simulink model "DCM_Controller_Due"  (R2020a)
settings: Solver=FixedStepAuto  StartTime=0.0  StopTime=inf  FixedStep=T  RelTol=1e-3  EnableMultiTasking=on
undefined symbols (not defined in the file): Iumax, Ki_I, Kp_I, Kp_W, Kphi, T, Ubat, wmax
libraries: arduinolib x7, eeStairGenerator x2
settings Model: SILPILModeSetting=veronly  ExtModeTrigDuration=2  Creator=Nguyen Tung  LastModifiedBy=Nguyen Tung
settings OptimizationCC: StrengthReduction=on  PassReuseOutputArgsAs=Individual arguments  ZeroExternalMemoryAtStartup=off  ZeroInternalMemoryAtStartup=off  MaxStackSize=64  OptimizeBlockOrder=speed  OptimizationPriority=Speed  OptimizationCustomize=off  MultiThreadedLoops=on  EfficientTunableParamExpr=on
settings DebuggingCC: ParameterTunabilityLossMsg=error
settings HardwareCC: ProdBitPerPointer=32  ProdBitPerSizeT=32  ProdBitPerPtrDiffT=32  ProdLargestAtomicInteger=Long  ProdLargestAtomicFloat=Double  ProdWordSize=32  ProdHWDeviceType=ARM Compatible->ARM Cortex
settings SFSimCC: MATLABDynamicMemAlloc=off
settings RTWCC: SystemTargetFile=ert.tlc  HardwareBoard=Arduino Due  TLCOptions=-aInlineSetEventsForThisBaseRateFcn=TLC_FALSE -aSuppressMultiTaskScheduler=TLC_FALSE -aRateBasedStepFcn=1  TemplateMakefile=ert_default_tmf  GenerateReport=on  Toolchain=Arduino ARM  BuildConfiguration=Faster Runs
settings CodeAppCC: ForceParamTrailComments=on  IgnoreCustomStorageClasses=off  OperatorAnnotations=on  SimulinkDataObjDesc=on  SFDataObjDesc=on  InsertBlockDesc=on
settings ERTTargetCC: SupportContinuousTime=on  SupportVariableSizeSignals=on  ExtModeStaticAllocSize=20000

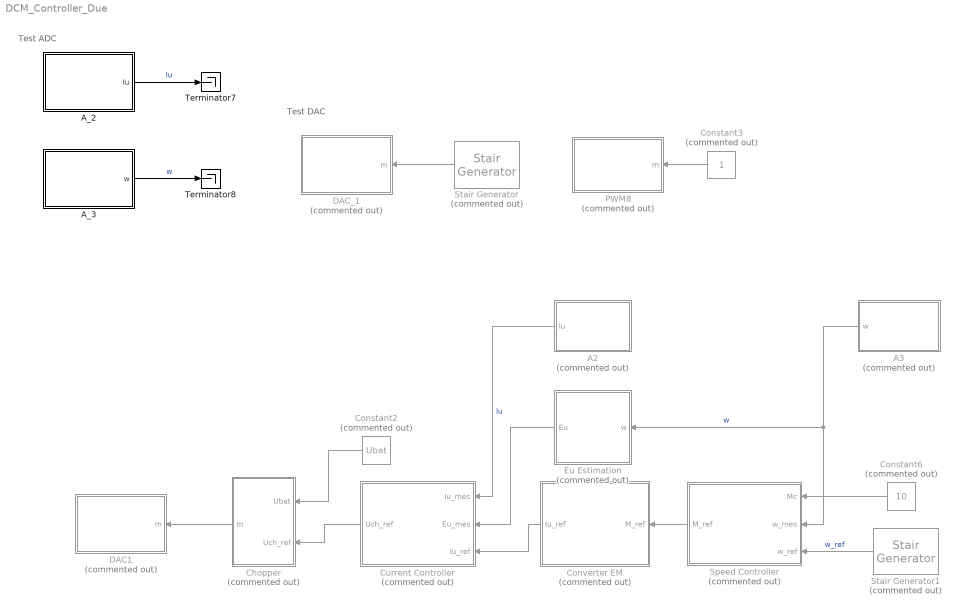
== system DCM_Controller_Due ==
  note: Test ADC
  note: Test DAC
  A2 : Subsystem  Commented=on
  A3 : Subsystem  Commented=on
  A_2 : Subsystem
  A_3 : Subsystem
  Chopper : Subsystem  Commented=on  AncestorBlock=simulink/SMC/Inversion EC avec mesure
      mask Display: plot(0,0,100,100,[10,30,90,70,10],[90,10,10,90,90])
  Constant2 : Constant  Commented=on  Value=Ubat
  Constant3 : Constant  Commented=on
  Constant6 : Constant  Commented=on  Value=10
  Converter EM : Subsystem  Commented=on  AncestorBlock=simulink/SMC/Inversion EC avec mesure
      mask Display: plot(0,0,100,100,[10,30,90,70,10],[90,10,10,90,90])
  Current Controller : Subsystem  Commented=on  AncestorBlock=simulink/SMC/Asservissement Correcteur IP
      mask Display: plot(0,0,100,100, [10,30,90,70,10,90],[90,10,10,90,90,10])
  DAC1 : Subsystem  Commented=on
  DAC_1 : Subsystem  Commented=on
  Eu Estimation : Subsystem  Commented=on  AncestorBlock=simulink/REM/EC EM
      mask Display: plot(0,0,100,100, 1.4*[50,57.68,60.77,63.08,64.97,66.58,68,69.26,70.4, 	71.42,72.36,78.28,80,78.28,72.36,71.42,70.4, 	69.26,68,66.58,64.97,63.08,60.77,57.68,50,42.32, 	39.23,36.92,35.03,33.42,32,30.74,29.6,28.58, 	27.64,21.72,20,21.72,27.64,28.58,29.6,30.74,32, 	33.42,35.03,36.92,39.23,42.32,50]-20, 1.4*[20,21,22,23,24,25,26,27,28,29,30,40,50,60,70,71,72, 	73,74,75,76,77,78,79,80,79,78,77,76,75,74,73,72, 	71,70,60,50,40,30,29,28,27,26,25,24,23,22,21,20]-20)
  PWM8 : Subsystem  Commented=on
  Speed Controller : Subsystem  Commented=on  AncestorBlock=simulink/SMC/Asservissement Correcteur IP
      mask Display: plot(0,0,100,100, [10,30,90,70,10,90],[90,10,10,90,90,10])
  Stair Generator : eeStairGenerator/Stair Generator  Commented=on  LabelModeActiveChoice=Discrete  TimeInput=[0 2 4 6 8 10 12]  AmplitudeInput=[0 0.2 0.4 0.6 0.8 1 0]  SampleTime=T  RepeatPattern=on  OutDataTypeStr=double
      settings: SourceProductBaseCode=PS
  Stair Generator1 : eeStairGenerator/Stair Generator  Commented=on  LabelModeActiveChoice=Discrete  TimeInput="[0 5  10  15  20 25 30 35 40 45]"  AmplitudeInput=[10 50 100 10 70 10 90 10 100 10]  SampleTime=T  RepeatPattern=on  OutDataTypeStr=double
      settings: SourceProductBaseCode=PS
  Terminator7 : Terminator
  Terminator8 : Terminator
  wires:
  Converter EM/1(Iu_ref) -> Current Controller/3(Iu_ref)
  A2/1(Iu) -> Current Controller/1(Iu_mes)  "Iu"
  Constant6/1 -> Speed Controller/1(Mc)
  Current Controller/1(Uch_ref) -> Chopper/2(Uch_ref)
  A3/1(w) -> Eu Estimation/1(w), Speed Controller/2(w_mes)  "w"
  Constant2/1 -> Chopper/1(Ubat)
  Speed Controller/1(M_ref) -> Converter EM/1(M_ref)
  Eu Estimation/1(Eu) -> Current Controller/2(Eu_mes)
  Stair Generator1/1 -> Speed Controller/3(w_ref)  "w_ref"
  Chopper/1(m) -> DAC1/1(m)
  Stair Generator/1 -> DAC_1/1(m)
  Constant3/1 -> PWM8/1(m)
  A_3/1(w) -> Terminator8/1  "w"
  A_2/1(Iu) -> Terminator7/1  "Iu"

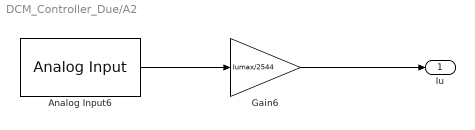
== system DCM_Controller_Due/A2 ==
  Analog Input6 : arduinolib/Analog Input  pinNumber=2  ReadResultsOnly=off  ConversionTriggerSource=Software  ExternalTriggerType=uint32( 0 )  OutputDataType=uint16  EnableConversionCompleteNotify=off  EnableOuputStatus=off  SampleTime=T  blockPlatform=arduino
  Gain6 : Gain  Gain=Iumax/2544
  Iu : Outport
  wires:
  Analog Input6/1 -> Gain6/1
  Gain6/1 -> Iu/1

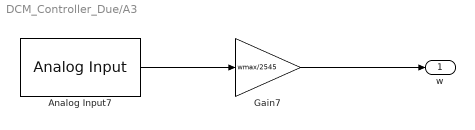
== system DCM_Controller_Due/A3 ==
  Analog Input7 : arduinolib/Analog Input  pinNumber=3  ReadResultsOnly=off  ConversionTriggerSource=Software  ExternalTriggerType=uint32( 0 )  OutputDataType=uint16  EnableConversionCompleteNotify=off  EnableOuputStatus=off  SampleTime=T  blockPlatform=arduino
  Gain7 : Gain  Gain=wmax/2545
  w : Outport
  wires:
  Analog Input7/1 -> Gain7/1
  Gain7/1 -> w/1

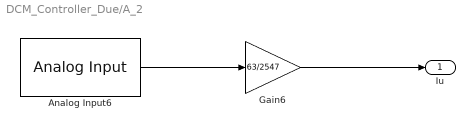
== system DCM_Controller_Due/A_2 ==
  Analog Input6 : arduinolib/Analog Input  pinNumber=2  ReadResultsOnly=off  ConversionTriggerSource=Software  ExternalTriggerType=uint32( 0 )  OutputDataType=uint16  EnableConversionCompleteNotify=off  EnableOuputStatus=off  SampleTime=T  blockPlatform=arduino
  Gain6 : Gain  Gain=63/2547
  Iu : Outport
  wires:
  Analog Input6/1 -> Gain6/1
  Gain6/1 -> Iu/1

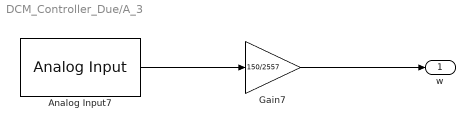
== system DCM_Controller_Due/A_3 ==
  Analog Input7 : arduinolib/Analog Input  pinNumber=3  ReadResultsOnly=off  ConversionTriggerSource=Software  ExternalTriggerType=uint32( 0 )  OutputDataType=uint16  EnableConversionCompleteNotify=off  EnableOuputStatus=off  SampleTime=T  blockPlatform=arduino
  Gain7 : Gain  Gain=150/2557
  w : Outport
  wires:
  Analog Input7/1 -> Gain7/1
  Gain7/1 -> w/1

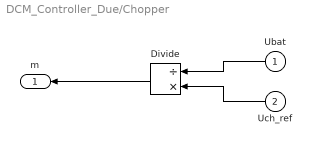
== system DCM_Controller_Due/Chopper ==
  Ubat : Inport
  Uch_ref : Inport  Port=2
  Divide : Product  Inputs=/*
  m : Outport
  wires:
  Ubat/1 -> Divide/1
  Uch_ref/1 -> Divide/2
  Divide/1 -> m/1

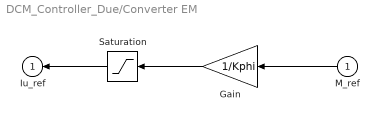
== system DCM_Controller_Due/Converter EM ==
  M_ref : Inport
  Gain : Gain  Gain=1/Kphi
  Saturation : Saturate  UpperLimit=Iumax  LowerLimit=0
  Iu_ref : Outport  InitialOutput=0  VectorParamsAs1DForOutWhenUnconnected=off
  wires:
  M_ref/1 -> Gain/1
  Gain/1 -> Saturation/1
  Saturation/1 -> Iu_ref/1

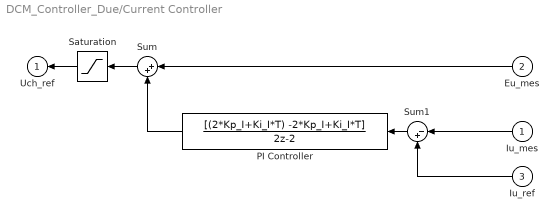
== system DCM_Controller_Due/Current Controller ==
  Iu_mes : Inport
  Eu_mes : Inport  Port=2
  Iu_ref : Inport  Port=3
  PI Controller : DiscreteTransferFcn  Numerator=[(2*Kp_I+Ki_I*T) -2*Kp_I+Ki_I*T]  Denominator=[2 -2]
  Saturation : Saturate  UpperLimit=Ubat  LowerLimit=0
  Sum : Sum  Inputs=|++
  Sum1 : Sum  Inputs=|-+
  Uch_ref : Outport  InitialOutput=0  VectorParamsAs1DForOutWhenUnconnected=off
  wires:
  Eu_mes/1 -> Sum/1
  Sum/1 -> Saturation/1
  Iu_mes/1 -> Sum1/1
  Sum1/1 -> PI Controller/1
  PI Controller/1 -> Sum/2
  Iu_ref/1 -> Sum1/2
  Saturation/1 -> Uch_ref/1

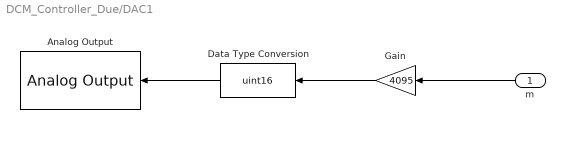
== system DCM_Controller_Due/DAC1 ==
  m : Inport
  Analog Output : arduinolib/Analog Output  DACpin=DAC1  blockPlatform=arduino
      settings: SourceProductBaseCode=ARDUINO
  Data Type Conversion : DataTypeConversion  OutDataTypeStr=uint16
  Gain : Gain  Gain=4095
  wires:
  m/1 -> Gain/1
  Gain/1 -> Data Type Conversion/1
  Data Type Conversion/1 -> Analog Output/1

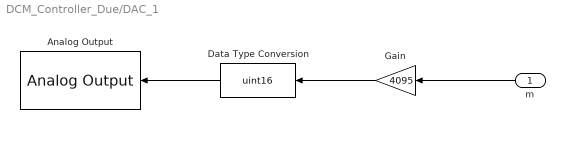
== system DCM_Controller_Due/DAC_1 ==
  m : Inport
  Analog Output : arduinolib/Analog Output  DACpin=DAC1  blockPlatform=arduino
      settings: SourceProductBaseCode=ARDUINO
  Data Type Conversion : DataTypeConversion  OutDataTypeStr=uint16
  Gain : Gain  Gain=4095
  wires:
  m/1 -> Gain/1
  Gain/1 -> Data Type Conversion/1
  Data Type Conversion/1 -> Analog Output/1

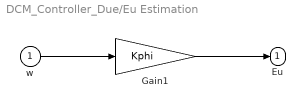
== system DCM_Controller_Due/Eu Estimation ==
  w : Inport
  Gain1 : Gain  Gain=Kphi
  Eu : Outport  InitialOutput=0  VectorParamsAs1DForOutWhenUnconnected=off
  wires:
  w/1 -> Gain1/1
  Gain1/1 -> Eu/1

== system DCM_Controller_Due/PWM8 ==
  m : Inport
  Gain : Gain  Gain=255
  PWM : arduinolib/PWM  pinNumber=8  frequencyType=Specify  desiredFrequency=1000  achievableFrequency=1000
  wires:
  Gain/1 -> PWM/1
  m/1 -> Gain/1

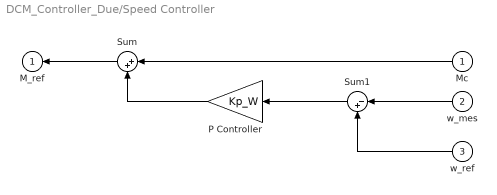
== system DCM_Controller_Due/Speed Controller ==
  Mc : Inport
  w_mes : Inport  Port=2
  w_ref : Inport  Port=3
  P Controller : Gain  Gain=Kp_W
  Sum : Sum  Inputs=|++
  Sum1 : Sum  Inputs=|-+
  M_ref : Outport  InitialOutput=0  VectorParamsAs1DForOutWhenUnconnected=off
  wires:
  Sum/1 -> M_ref/1
  w_ref/1 -> Sum1/2
  Sum1/1 -> P Controller/1
  P Controller/1 -> Sum/2
  Mc/1 -> Sum/1
  w_mes/1 -> Sum1/1
